simulink model "Expriment_Emotion"  (R2014a)
settings: Solver=FixedStepDiscrete  SolverMode=SingleTasking  StartTime=0.0  StopTime=inf  FixedStep=0.01  RelTol=1e-3
PostLoadFcn:
  | h_RPStest = RPStest;
model workspace (MAT data in the model file):
  gtest = 0
undefined symbols (not defined in the file or in its folder): avert, avert_freq_factor, avert_gaze_dirs_chance, avert_gaze_duration_factor, avert_head_frequency_factor, avert_head_speed, BML, BML1, BML2, bmlsL, bmlsM, bodyBusyFlag, clock, emotion_amount_factor, faceBusyFlag, fileID, GAZE_WIN, gazing, mut_freq_factor, mutual_gaze_duration_factor, P, pose_cat_chance, pose_chanc_factor, pose_chance_factor, pose_frequency_factor, pose_lean, pose_lean_flag, pose_space, pose_speed, pose_twitch, pr, serial, STATE_BEFORE, STATE_GO, STATE_OVER, STATE_READY, Stateflow
libraries: simulink x24, instrumentlib x6, realtime_pacer_lib x2, lib_affectiveChar_behavior x1, lib_affectiveChar_input x1
(part 6 of 6)

== matlab function Expriment_Emotion/facialExpr/facialExprGen/emotionBMLsLoop/loopInBmls ==
  data: i input double size=1 [1..]; arrAU input; eAmount input; arrBML output
function arrBML = fcn(i,arrAU,eAmount)
    %#codegen
    coder.extrinsic('sprintf');
    coder.extrinsic('strcat');
    
    %Maryam, 14-10-2015
    %'strcat' dimension 2  maximum size is 453,it was not possible to concat and send all bmls 
    %for one emotion together(used simulink for loop )    
    
    AU=arrAU(i);eA=eAmount(i);   
    c1 = countDigits(AU);c2 = countDigits(eA);

    str1 = sprintf('<?xml version=\"1.0\" ?><act><bml>');
    
    if(max(ceil(log10(abs(AU))),1)==1) %if AU is one-digit
        temp = sprintf('<face type=\"FACS\" side=\"BOTH\" au=\"%1d\"  start=\"0\" end=\"3\" amount=\"%0.1f\"/>',AU,eA); 
        temp2=strcat(str1,temp);
        str1=temp2;
    else      
        temp = sprintf('<face type=\"FACS\" side=\"BOTH\" au=\"%2d\"  start=\"0\" end=\"3\" amount=\"%0.1f\"/>',AU,eA);
        temp2=strcat(str1,temp);
        str1=temp2;
    end

    str2 = sprintf('</bml></act>');
    %n=length(arrAU);
    %mystr=blanks(arrAU(n));
    mystr=blanks(140+c1+c2);
    mystr = strcat (str1,str2);    
    arrBML = encStr2Arr(mystr);

== matlab function Expriment_Emotion/facialExpr/facialExprGen/forloop/makeBmlsFor ==
  data: i input double size=1 [1..]; arrAU input; eAmount input; arrBML1 output; arrBML2 output; arrBML3 output; arrBML4 output; arrBML5 output; arrBML6 output
function [arrBML1,arrBML2,arrBML3,arrBML4,arrBML5,arrBML6] = fcn(i,arrAU,eAmount)
    %#codegen
    coder.extrinsic('sprintf');
    coder.extrinsic('strcat');
    arrBML1=encStr2Arr('');arrBML2=encStr2Arr('');arrBML3=encStr2Arr('');
    arrBML4=encStr2Arr('');arrBML5=encStr2Arr('');arrBML6=encStr2Arr('');
    %Maryam, 14-10-2015
    %'strcat' dimension 2  maximum size is 453,it was not possible to concat and send all bmls 
    %for one emotion together(used simulink for loop )    
    
    AU=arrAU(i);eA=eAmount(i);   
    c1 = countDigits(AU);c2 = countDigits(eA);

    str1 = sprintf('<?xml version=\"1.0\" ?><act><bml>');
    
    if(max(ceil(log10(abs(AU))),1)==1) %if AU is one-digit
        temp = sprintf('<face type=\"FACS\" side=\"BOTH\" au=\"%1d\"  start=\"0\" ready=\"1\" stroke=\"2\"  relax=\"3\" end=\"4\" amount=\"%0.1f\"/>',AU,eA); 
        temp2=strcat(str1,temp);
        str1=temp2;
    else      
        temp = sprintf('<face type=\"FACS\" side=\"BOTH\" au=\"%2d\" start=\"0\" ready=\"1\" stroke=\"2\"  relax=\"3\" end=\"4\" amount=\"%0.1f\"/>',AU,eA);
        temp2=strcat(str1,temp);
        str1=temp2;
    end

    str2 = sprintf('</bml></act>');
    %n=length(arrAU);
    %mystr=blanks(arrAU(n));
    mystr=blanks(140+c1+c2);
    mystr = strcat (str1,str2);  
    if(i==1)
        arrBML1 = encStr2Arr(mystr);
    elseif(i==2)
        arrBML2 = encStr2Arr(mystr);
     elseif(i==3)
            arrBML3 = encStr2Arr(mystr);
     elseif(i==4)
            arrBML4 = encStr2Arr(mystr);
     elseif(i==5)
            arrBML5 = encStr2Arr(mystr);
     elseif(i==6)
            arrBML6 = encStr2Arr(mystr);
    end

== matlab function Expriment_Emotion/facialExpr/facialExprGen/matlabFuncIf/reset ==
  data: L input; u1 input; y output
function y = fcn(L,u1)
if(u1<=L)
    y= u1;
else
    y =1;
end

== matlab function Expriment_Emotion/facialExpr/facialExprGen/matlabFuncIf/displayBMLs ==
  data: e input; l input; i input double size=1 [1..]; bml input
function fcn(e,l,i,bml)
%#codegen
fprintf('%s','e:');fprintf('%f',e);
fprintf('%s','  ,L:');fprintf('%f',l);
fprintf('%s','  ,i:');fprintf('%f',i);
disp(decArr2Str(bml));

== matlab function Expriment_Emotion/facialExpr/facialExprGen/matlabFuncIf/plusOne ==
  data: y output; i input double size=1
function y  = iCheck(i)
%#codegen
    y=i+1;

== matlab function Expriment_Emotion/facialExpr/facialExprGen/matlabFuncIf/makeBmls ==
  data: i input double size=1 [1..]; arrAU input; eAmount input; arrBML output
function arrBML = fcn(i,arrAU,eAmount)
    %#codegen
    coder.extrinsic('sprintf');
    coder.extrinsic('strcat');
    
    %Maryam, 14-10-2015
    %'strcat' dimension 2  maximum size is 453,it was not possible to concat and send all bmls 
    %for one emotion together(used simulink for loop )    
    
    AU=arrAU(i);eA=eAmount(i);   
    c1 = countDigits(AU);c2 = countDigits(eA);

    str1 = sprintf('<?xml version=\"1.0\" ?><act><bml>');
    
    if(max(ceil(log10(abs(AU))),1)==1) %if AU is one-digit
        temp = sprintf('<face type=\"FACS\" side=\"BOTH\" au=\"%1d\"  start=\"0\" ready=\"1\" stroke=\"2\"  relax=\"300\" end=\"400\" amount=\"%0.1f\"/>',AU,eA); 
        temp2=strcat(str1,temp);
        str1=temp2;
    else      
        temp = sprintf('<face type=\"FACS\" side=\"BOTH\" au=\"%2d\" start=\"0\" ready=\"1\" stroke=\"2\"  relax=\"300\" end=\"400\" amount=\"%0.1f\"/>',AU,eA);
        temp2=strcat(str1,temp);
        str1=temp2;
    end

    str2 = sprintf('</bml></act>');
    %n=length(arrAU);
    %mystr=blanks(arrAU(n));
    mystr=blanks(142+c1+c2);
    mystr = strcat (str1,str2);    
    arrBML = encStr2Arr(mystr);

== matlab function Expriment_Emotion/facialExpr/facialExprGen/forloop1/displayBMLs ==
  data: e input; l input; i input double size=1 [1..]; bml input
function fcn(e,l,i,bml)
%#codegen
fprintf('%s','e:');fprintf('%f',e);
fprintf('%s','  ,L:');fprintf('%f',l);
fprintf('%s','  ,i:');fprintf('%f',i);
disp(decArr2Str(bml));

== matlab function Expriment_Emotion/facialExpr/facialExprGen/forloop1/makeBmls ==
  data: i input double size=1 [1..]; arrAU input; eAmount input; arrBML output
function arrBML = fcn(i,arrAU,eAmount)
    %#codegen
    coder.extrinsic('sprintf');
    coder.extrinsic('strcat');
    
    %Maryam, 14-10-2015
    %'strcat' dimension 2  maximum size is 453,it was not possible to concat and send all bmls 
    %for one emotion together(used simulink for loop )    
    
    AU=arrAU(i);eA=eAmount(i);   
    c1 = countDigits(AU);c2 = countDigits(eA);

    str1 = sprintf('<?xml version=\"1.0\" ?><act><bml>');
    
    if(max(ceil(log10(abs(AU))),1)==1) %if AU is one-digit
        temp = sprintf('<face type=\"FACS\" side=\"BOTH\" au=\"%1d\"  start=\"0\" ready=\"1\" stroke=\"2\"  relax=\"3\" end=\"4\" amount=\"%0.1f\"/>',AU,eA); 
        temp2=strcat(str1,temp);
        str1=temp2;
    else      
        temp = sprintf('<face type=\"FACS\" side=\"BOTH\" au=\"%2d\" start=\"0\" ready=\"1\" stroke=\"2\"  relax=\"3\" end=\"4\" amount=\"%0.1f\"/>',AU,eA);
        temp2=strcat(str1,temp);
        str1=temp2;
    end

    str2 = sprintf('</bml></act>');
    %n=length(arrAU);
    %mystr=blanks(arrAU(n));
    mystr=blanks(140+c1+c2);
    mystr = strcat (str1,str2);    
    arrBML = encStr2Arr(mystr);

== stateflow chart Expriment_Emotion/GazeFollowSubsystem/resetGazeTarget/createGazePawn ==
  state sendSBM(In2) [function]
  state stateCreatePawn
    entry:
    sendSBM(encStr2Arr('scene.getPawn(\"gazeTarget\").setPosition(SrVec(0,1.6,10))'));
  (default) -> stateCreatePawn
  data: In2 function_input double size=[1000 1]

== matlab function Expriment_Emotion/chack_E_Change1/checkNeutral ==
  data: notNeutral output double size=1; e input
function notNeutral = fcn(e)
%#codegen

if(e~=6)
    notNeutral=1;
else
    notNeutral=0;
end

== matlab function Expriment_Emotion/setPersonality ==
  data: extrovert input; personality output; neurotic input
function personality = fcn(extrovert,neurotic)
%#codegen
% 1 HEHN 2 LEHN 3 HELN 4 LELN
if(extrovert==1)
    if(neurotic==1)
        personality = 1;% 1 HEHN
    else 
        personality = 3;%HELN
    end
else
    if(neurotic==1)
        personality = 2;%LEHN
    else
        personality = 4;%LELN
    end
end

== matlab function Expriment_Emotion/EmotionSubsystem/calculateValenceArousal/HEHN_VA_Emo ==
  data: V input; e output double size=1; A input double
function e = fcn(V, A)

aVarTruthTableCondition_1 = false;
aVarTruthTableCondition_2 = false;
aVarTruthTableCondition_3 = false;
aVarTruthTableCondition_4 = false;
aVarTruthTableCondition_5 = false;
aVarTruthTableCondition_6 = false;
aVarTruthTableCondition_7 = false;
aVarTruthTableCondition_8 = false;


% 7-happy  2,1

aVarTruthTableCondition_1 = logical(V>10 && A<40 && A>10);

% 8-ex  1,2 AND 2,2

aVarTruthTableCondition_2 = logical(V>0 && A>40);

% 4-fear  -1,2 AND -2,2

aVarTruthTableCondition_3 = logical(V<0 && A>40);

% 3-frust  -2,1

aVarTruthTableCondition_4 = logical(V<-10 && A<40 && A>10);

% 6-pleased  2,-1

aVarTruthTableCondition_5 = logical(V>10 && A<-10 && A>-40);

% 5-calm  1,-2 AND 2,-2

aVarTruthTableCondition_6 = logical(V>0 && A<-40);

% 1-bored  -1,-2 AND -2,-2

aVarTruthTableCondition_7 = logical(V<0 && A<-40);

% 2-sad  -2,-1

aVarTruthTableCondition_8 = logical(V<-10 && A<-10 && A>-40);

if (aVarTruthTableCondition_1)
    aFcnTruthTableAction_1();
elseif (aVarTruthTableCondition_2)
    aFcnTruthTableAction_2();
elseif (aVarTruthTableCondition_3)
    aFcnTruthTableAction_3();
elseif (aVarTruthTableCondition_4)
    aFcnTruthTableAction_4();
elseif (aVarTruthTableCondition_5)
    aFcnTruthTableAction_5();
elseif (aVarTruthTableCondition_6)
    aFcnTruthTableAction_6();
elseif (aVarTruthTableCondition_7)
    aFcnTruthTableAction_7();
elseif (aVarTruthTableCondition_8)
    aFcnTruthTableAction_8();
else % Default
    aFcnTruthTableAction_5();
end

function aFcnTruthTableAction_1()

% happy

e=7;

function aFcnTruthTableAction_2()

% excited

e=8;

function aFcnTruthTableAction_3()

% fear

e=4;

function aFcnTruthTableAction_4()

% frustration

e=3;

function aFcnTruthTableAction_5()

% pleased

e=6;

function aFcnTruthTableAction_6()

% contempt

e=5;

function aFcnTruthTableAction_7()

% bored

e=1;

function aFcnTruthTableAction_8()

% sad

e=2;

== matlab function Expriment_Emotion/EmotionSubsystem/calculateValenceArousal/HELN_VA_Emo ==
  data: V input; e output double size=1; A input double
function e = fcn(V, A)

aVarTruthTableCondition_1 = false;
aVarTruthTableCondition_2 = false;
aVarTruthTableCondition_3 = false;
aVarTruthTableCondition_4 = false;
aVarTruthTableCondition_5 = false;
aVarTruthTableCondition_6 = false;
aVarTruthTableCondition_7 = false;
aVarTruthTableCondition_8 = false;


% 7-happy  2,1

aVarTruthTableCondition_1 = logical(V>10 && A<40 && A>10);

% 8-ex  1,2 AND 2,2

aVarTruthTableCondition_2 = logical(V>0 && A>40);

% 4-fear  -1,2 AND -2,2

aVarTruthTableCondition_3 = logical(V<0 && A>40);

% 3-frust  -2,1

aVarTruthTableCondition_4 = logical(V<-10 && A<40 && A>10);

% 6-idle  2,-1

aVarTruthTableCondition_5 = logical(V>10 && A<-10 && A>-40);

% 5-calm  1,-2 AND 2,-2

aVarTruthTableCondition_6 = logical(V>0 && A<-40);

% 1-bored  -1,-2 AND -2,-2

aVarTruthTableCondition_7 = logical(V<0 && A<-40);

% 2-sad  -2,-1

aVarTruthTableCondition_8 = logical(V<-10 && A<-10 && A>-40);

if (aVarTruthTableCondition_1)
    aFcnTruthTableAction_1();
elseif (aVarTruthTableCondition_2)
    aFcnTruthTableAction_2();
elseif (aVarTruthTableCondition_3)
    aFcnTruthTableAction_3();
elseif (aVarTruthTableCondition_4)
    aFcnTruthTableAction_4();
elseif (aVarTruthTableCondition_5)
    aFcnTruthTableAction_5();
elseif (aVarTruthTableCondition_6)
    aFcnTruthTableAction_6();
elseif (aVarTruthTableCondition_7)
    aFcnTruthTableAction_7();
elseif (aVarTruthTableCondition_8)
    aFcnTruthTableAction_8();
else % Default
    aFcnTruthTableAction_5();
end

function aFcnTruthTableAction_1()

% happy

e=7;

function aFcnTruthTableAction_2()

% excited

e=8;

function aFcnTruthTableAction_3()

% fear

e=4;

function aFcnTruthTableAction_4()

% frustration

e=3;

function aFcnTruthTableAction_5()

% idle

e=6;

function aFcnTruthTableAction_6()

% contempt

e=5;

function aFcnTruthTableAction_7()

% bored

e=1;

function aFcnTruthTableAction_8()

% sad

e=2;

== matlab function Expriment_Emotion/gazeInputArray/makeGazeArray ==
  data: r1 input; y output double size=[1,6]; r2 input; r3 input; r4 input; r5 input; r6 input
function y = fcn(r1,r2,r3,r4,r5,r6)
%#codegen
y=[0,0,0,0,0,0];
y(:,1) = floor(r1);
y(:,2) = floor(r2);
y(:,3) = floor(r3);
y(:,4) = floor(r4);
y(:,5) = floor(r5);
y(:,6) = floor(r6);

== matlab function Expriment_Emotion/EmotionSubsystem/calculateValenceArousal/LELN_VA_Emo ==
  data: V input; e output double size=1; A input double
function e = fcn(V, A)

aVarTruthTableCondition_1 = false;
aVarTruthTableCondition_2 = false;
aVarTruthTableCondition_3 = false;
aVarTruthTableCondition_4 = false;
aVarTruthTableCondition_5 = false;
aVarTruthTableCondition_6 = false;
aVarTruthTableCondition_7 = false;
aVarTruthTableCondition_8 = false;


% 7-happy  2,1

aVarTruthTableCondition_1 = logical(V>20 && A<40 && A>20);

% 8-ex  1,2 AND 2,2

aVarTruthTableCondition_2 = logical(V>0 && A>40);

% 4-fear  -1,2 AND -2,2

aVarTruthTableCondition_3 = logical(V<0 && A>40);

% 3-frust  -2,1

aVarTruthTableCondition_4 = logical(V<-20 && A<40 && A>20);

% 6-idle  2,-1

aVarTruthTableCondition_5 = logical(V>20 && A<-20 && A>-40);

% 5-calm  1,-2 AND 2,-2

aVarTruthTableCondition_6 = logical(V>0 && A<-40);

% 1-bored  -1,-2 AND -2,-2

aVarTruthTableCondition_7 = logical(V<0 && A<-40);

% 2-sad  -2,-1

aVarTruthTableCondition_8 = logical(V<-20 && A<-20 && A>-40);

if (aVarTruthTableCondition_1)
    aFcnTruthTableAction_1();
elseif (aVarTruthTableCondition_2)
    aFcnTruthTableAction_2();
elseif (aVarTruthTableCondition_3)
    aFcnTruthTableAction_3();
elseif (aVarTruthTableCondition_4)
    aFcnTruthTableAction_4();
elseif (aVarTruthTableCondition_5)
    aFcnTruthTableAction_5();
elseif (aVarTruthTableCondition_6)
    aFcnTruthTableAction_6();
elseif (aVarTruthTableCondition_7)
    aFcnTruthTableAction_7();
elseif (aVarTruthTableCondition_8)
    aFcnTruthTableAction_8();
else % Default
    aFcnTruthTableAction_5();
end

function aFcnTruthTableAction_1()

% happy

e=7;

function aFcnTruthTableAction_2()

% excited

e=8;

function aFcnTruthTableAction_3()

% fear

e=4;

function aFcnTruthTableAction_4()

% frustration

e=3;

function aFcnTruthTableAction_5()

% idle

e=6;

function aFcnTruthTableAction_6()

% contempt

e=5;

function aFcnTruthTableAction_7()

% bored

e=1;

function aFcnTruthTableAction_8()

% sad

e=2;

== matlab function Expriment_Emotion/EmotionSubsystem/calculateValenceArousal/HEHN_A ==
  data: a2 output double size=1; a1 input double size=1
function a2 = fcn(a1)

aVarTruthTableCondition_1 = false;
aVarTruthTableCondition_2 = false;



aVarTruthTableCondition_1 = logical(a1>10);


aVarTruthTableCondition_2 = logical(a1<-10);

if (aVarTruthTableCondition_1)
    aFcnTruthTableAction_1();
elseif (aVarTruthTableCondition_2)
    aFcnTruthTableAction_2();
else % Default
    aFcnTruthTableAction_3();
end

function aFcnTruthTableAction_1()


a2=a1;

function aFcnTruthTableAction_2()


a2=a1;

function aFcnTruthTableAction_3()


a2=0;

== matlab function Expriment_Emotion/EmotionSubsystem/calculateValenceArousal/LEHN_A ==
  data: a2 output double size=1; a1 input double size=1
function a2 = fcn(a1)

aVarTruthTableCondition_1 = false;
aVarTruthTableCondition_2 = false;



aVarTruthTableCondition_1 = logical(a1>25);


aVarTruthTableCondition_2 = logical(a1<-25);

if (aVarTruthTableCondition_1)
    aFcnTruthTableAction_1();
elseif (aVarTruthTableCondition_2)
    aFcnTruthTableAction_2();
else % Default
    aFcnTruthTableAction_3();
end

function aFcnTruthTableAction_1()


a2=a1;

function aFcnTruthTableAction_2()


a2=a1;

function aFcnTruthTableAction_3()


a2=0;

== matlab function Expriment_Emotion/EmotionSubsystem/calculateValenceArousal/HELN_A ==
  data: a2 output double size=1; a1 input double size=1
function a2 = fcn(a1)

aVarTruthTableCondition_1 = false;
aVarTruthTableCondition_2 = false;



aVarTruthTableCondition_1 = logical(a1>10);


aVarTruthTableCondition_2 = logical(a1<-10);

if (aVarTruthTableCondition_1)
    aFcnTruthTableAction_1();
elseif (aVarTruthTableCondition_2)
    aFcnTruthTableAction_2();
else % Default
    aFcnTruthTableAction_3();
end

function aFcnTruthTableAction_1()


a2=a1;

function aFcnTruthTableAction_2()


a2=a1;

function aFcnTruthTableAction_3()


a2=0;

== matlab function Expriment_Emotion/poseInputArray/makePoseArray ==
  data: r1 input; y output double size=[1,6]; r2 input; r3 input; r4 input; r5 input; r6 input
function y = fcn(r1,r2,r3,r4,r5,r6)
%#codegen
y=[0,0,0,0,0,0];
y(:,1) = floor(r1);
y(:,2) = floor(r2);
y(:,3) = floor(r3);
y(:,4) = floor(r4);
y(:,5) = floor(r5);
y(:,6) = floor(r6);

== matlab function Expriment_Emotion/EmotionSubsystem/calculateValenceArousal/HEHN plot ==
  data: v input; a input
function fcn(v,a)
%coder.extrinsic to bypass code generation
coder.extrinsic('fscanf')
coder.extrinsic('get_param');
% coder.extrinsic('importdata');

currentTime=get_param('Expriment_FacialExpr','SimulationTime');%use name of simulink proj

A = [v;a;currentTime];
fileID = fopen('HEHN_VA_table.txt','a');
fprintf(fileID,'%0.1f,%0.1f,%0.1f\r\n',A);
fclose(fileID);

% matrix = importdata('HEHN_VA_table.txt',','); 
% tri = delaunay(matrix(:,1),matrix(:,2));
% trisurf(tri,matrix(:,1),matrix(:,2),matrix(:,3))
% shading interp
% colorbar

%-----------------------------------------
% fileID = fopen('HEHN_VA_table.txt','r');
% formatSpec = '%1f\r %1f\r %1f\r\n';
% sizeA = [3 Inf];
% A = fscanf(fileID,formatSpec,sizeA)
% % A = A'
% fclose(fileID);

% x = zeros(100,2);y = zeros(100,2);
% filename = 'HEHN_VA_table.txt';
% delimiterIn = ' ';
% headerlinesIn = 1;
% A = importdata(filename,delimiterIn,headerlinesIn);

% fileID=fopen('HEHN_VA_table4.txt');
% s=textscan(fileID,'%d %d %d','headerlines',23);
% fclose(fileID);
% x=s{1}

== matlab function Expriment_Emotion/EmotionSubsystem/calculateValenceArousal/LEHN plot ==
  data: v input; a input
function fcn(v,a)
%coder.extrinsic to bypass code generation
coder.extrinsic('fscanf')
coder.extrinsic('get_param');
% coder.extrinsic('importdata');

currentTime=get_param('Expriment_FacialExpr','SimulationTime');%use name of simulink proj

A = [v;a;currentTime];

fileID = fopen('LEHN_VA_table.txt','a');
fprintf(fileID,'%0.1f,%0.1f,%0.1f\r\n',A);
fclose(fileID);

%use the following to draw the plot
%tmp_data = importdata('HEHN_VA_table.txt',','); 
%no need: x=tmp_data(:,1);y=tmp_data(:,2);z=tmp_data(:,3)
%matrix=tmp_data
%tri = delaunay(matrix(:,1),matrix(:,2));
%trisurf(tri,matrix(:,1),matrix(:,2),matrix(:,3))
%shading interp

%-----------------------------------------
% fileID = fopen('HEHN_VA_table.txt','r');
% formatSpec = '%1f\r %1f\r %1f\r\n';
% sizeA = [3 Inf];
% A = fscanf(fileID,formatSpec,sizeA)
% % A = A'
% fclose(fileID);

% x = zeros(100,2);y = zeros(100,2);
% filename = 'HEHN_VA_table.txt';
% delimiterIn = ' ';
% headerlinesIn = 1;
% A = importdata(filename,delimiterIn,headerlinesIn);

% fileID=fopen('HEHN_VA_table4.txt');
% s=textscan(fileID,'%d %d %d','headerlines',23);
% fclose(fileID);
% x=s{1}

== matlab function Expriment_Emotion/EmotionSubsystem/calculateValenceArousal/HELN plot ==
  data: v input; a input
function fcn(v,a)
%coder.extrinsic to bypass code generation
coder.extrinsic('fscanf')
coder.extrinsic('get_param');
% coder.extrinsic('importdata');

currentTime=get_param('Expriment_FacialExpr','SimulationTime');%use name of simulink proj

A = [v;a;currentTime];

fileID = fopen('HELN_VA_table.txt','a');
fprintf(fileID,'%0.1f,%0.1f,%0.1f\r\n',A);
fclose(fileID);

%use the following to draw the plot
%tmp_data = importdata('HEHN_VA_table.txt',','); 
%no need: x=tmp_data(:,1);y=tmp_data(:,2);z=tmp_data(:,3)
%matrix=tmp_data
%tri = delaunay(matrix(:,1),matrix(:,2));
%trisurf(tri,matrix(:,1),matrix(:,2),matrix(:,3))
%shading interp

%-----------------------------------------
% fileID = fopen('HEHN_VA_table.txt','r');
% formatSpec = '%1f\r %1f\r %1f\r\n';
% sizeA = [3 Inf];
% A = fscanf(fileID,formatSpec,sizeA)
% % A = A'
% fclose(fileID);

% x = zeros(100,2);y = zeros(100,2);
% filename = 'HEHN_VA_table.txt';
% delimiterIn = ' ';
% headerlinesIn = 1;
% A = importdata(filename,delimiterIn,headerlinesIn);

% fileID=fopen('HEHN_VA_table4.txt');
% s=textscan(fileID,'%d %d %d','headerlines',23);
% fclose(fileID);
% x=s{1}

== matlab function Expriment_Emotion/EmotionSubsystem/calculateValenceArousal/LELN plot ==
  data: v input; a input
function fcn(v,a)
%coder.extrinsic to bypass code generation
coder.extrinsic('fscanf')
coder.extrinsic('get_param');
% coder.extrinsic('importdata');

currentTime=get_param('Expriment_FacialExpr','SimulationTime');%use name of simulink proj

A = [v;a;currentTime];

fileID = fopen('LELN_VA_table.txt','a');
fprintf(fileID,'%0.1f,%0.1f,%0.1f\r\n',A);
fclose(fileID);

%use the following to draw the plot
%matrix = importdata('HEHN_VA_table.txt',','); 
%tri = delaunay(matrix(:,1),matrix(:,2));
%trisurf(tri,matrix(:,1),matrix(:,2),matrix(:,3))
%shading interp
%colorbar
%-----------------------------------------
% fileID = fopen('HEHN_VA_table.txt','r');
% formatSpec = '%1f\r %1f\r %1f\r\n';
% sizeA = [3 Inf];
% A = fscanf(fileID,formatSpec,sizeA)
% % A = A'
% fclose(fileID);

% x = zeros(100,2);y = zeros(100,2);
% filename = 'HEHN_VA_table.txt';
% delimiterIn = ' ';
% headerlinesIn = 1;
% A = importdata(filename,delimiterIn,headerlinesIn);

% fileID=fopen('HEHN_VA_table4.txt');
% s=textscan(fileID,'%d %d %d','headerlines',23);
% fclose(fileID);
% x=s{1}

== matlab function Expriment_Emotion/EmotionSubsystem/calculateValenceArousal/LELN_A ==
  data: a2 output double size=1; a1 input double size=1
function a2 = fcn(a1)

aVarTruthTableCondition_1 = false;
aVarTruthTableCondition_2 = false;



aVarTruthTableCondition_1 = logical(a1>25);


aVarTruthTableCondition_2 = logical(a1<-25);

if (aVarTruthTableCondition_1)
    aFcnTruthTableAction_1();
elseif (aVarTruthTableCondition_2)
    aFcnTruthTableAction_2();
else % Default
    aFcnTruthTableAction_3();
end

function aFcnTruthTableAction_1()


a2=a1;

function aFcnTruthTableAction_2()


a2=a1;

function aFcnTruthTableAction_3()


a2=0;

== matlab function Expriment_Emotion/EmotionSubsystem/calculateValenceArousal/HEHN_V ==
  data: v2 output double size=1; v1 input double size=1
function v2 = fcn(v1)

aVarTruthTableCondition_1 = false;
aVarTruthTableCondition_2 = false;



aVarTruthTableCondition_1 = logical(v1>10);


aVarTruthTableCondition_2 = logical(v1<-10);

if (aVarTruthTableCondition_1)
    aFcnTruthTableAction_1();
elseif (aVarTruthTableCondition_2)
    aFcnTruthTableAction_2();
else % Default
    aFcnTruthTableAction_3();
end

function aFcnTruthTableAction_1()


v2=v1;

function aFcnTruthTableAction_2()


v2=v1;

function aFcnTruthTableAction_3()


v2=0;

== matlab function Expriment_Emotion/EmotionSubsystem/calculateValenceArousal/LEHN_V ==
  data: v2 output double size=1; v1 input double size=1
function v2 = fcn(v1)

aVarTruthTableCondition_1 = false;
aVarTruthTableCondition_2 = false;



aVarTruthTableCondition_1 = logical(v1>25);


aVarTruthTableCondition_2 = logical(v1<-25);

if (aVarTruthTableCondition_1)
    aFcnTruthTableAction_1();
elseif (aVarTruthTableCondition_2)
    aFcnTruthTableAction_2();
else % Default
    aFcnTruthTableAction_3();
end

function aFcnTruthTableAction_1()


v2=v1;

function aFcnTruthTableAction_2()


v2=v1;

function aFcnTruthTableAction_3()


v2=0;

== matlab function Expriment_Emotion/EmotionSubsystem/calculateValenceArousal/HELN_V ==
  data: v2 output double size=1; v1 input double size=1
function v2 = fcn(v1)

aVarTruthTableCondition_1 = false;
aVarTruthTableCondition_2 = false;



aVarTruthTableCondition_1 = logical(v1>10);


aVarTruthTableCondition_2 = logical(v1<-10);

if (aVarTruthTableCondition_1)
    aFcnTruthTableAction_1();
elseif (aVarTruthTableCondition_2)
    aFcnTruthTableAction_2();
else % Default
    aFcnTruthTableAction_3();
end

function aFcnTruthTableAction_1()


v2=v1;

function aFcnTruthTableAction_2()


v2=v1;

function aFcnTruthTableAction_3()


v2=0;

== matlab function Expriment_Emotion/EmotionSubsystem/calculateValenceArousal/LELN_V ==
  data: v2 output double size=1; v1 input double size=1
function v2 = fcn(v1)

aVarTruthTableCondition_1 = false;
aVarTruthTableCondition_2 = false;



aVarTruthTableCondition_1 = logical(v1>25);


aVarTruthTableCondition_2 = logical(v1<-25);

if (aVarTruthTableCondition_1)
    aFcnTruthTableAction_1();
elseif (aVarTruthTableCondition_2)
    aFcnTruthTableAction_2();
else % Default
    aFcnTruthTableAction_3();
end

function aFcnTruthTableAction_1()


v2=v1;

function aFcnTruthTableAction_2()


v2=v1;

function aFcnTruthTableAction_3()


v2=0;

== stateflow chart Expriment_Emotion/CharacterControl/emotion_Behavior_Factors ==
  state init
    entry: mutual_gaze_duration_factor=1;avert_gaze_duration_factor=1;avert_head_frequency_factor=20;avert_head_speed=1;avert_gaze_dirs_chance=0;,avert_freq_factor=1;mut_freq_factor=1;
    pose_frequency_factor=20;pose_chanc_factor=1;pose_cat_chance=70;pose_lean=12;pose_speed=1;pose_lean_flag=0;pose_space=0;
  state wait
  state setBehavior
    entry:
    [mutual_gaze_duration_factor, avert_gaze_duration_factor,avert_head_frequency_factor,avert_head_speed,avert_gaze_dirs_chance,avert_freq_factor,mut_freq_factor]=sharedFunc.setGazeFactors(inV,inA,personality,personalityFlag,vaFlag,gazeArray);
    [pose_twitch,pose_frequency_factor,pose_chanc_factor,pose_cat_chance,pose_lean,pose_speed,pose_lean_flag,pose_space]=sharedFunc.setPoseFactors(inV,inA,personality,personalityFlag,vaFlag,poseArray,personalityChange);
  state sharedFunc [group]
  (default) -> init
  init -> wait
  wait -> setBehavior [order 2] : [vChange==1]
  wait -> setBehavior [order 1] : [aChange==1]
  setBehavior -> wait
  data: inA input double size=1; inV input double size=1; personality input; gazeArray input; aChange input; personalityFlag input; vaFlag input; avert_head_frequency_factor data_store_memory; avert_gaze_duration_factor data_store_memory; mutual_gaze_duration_factor data_store_memory; avert_head_speed data_store_memory; avert_gaze_dirs_chance data_store_memory; poseArray input; pose_lean data_store_memory; pose_speed data_store_memory; pose_lean_flag data_store_memory; pose_cat_chance data_store_memory; pose_frequency_factor data_store_memory; pose_chanc_factor data_store_memory; personalityChange input; avert_freq_factor data_store_memory; mut_freq_factor data_store_memory; pose_twitch data_store_memory; vChange input; pose_space data_store_memory

== matlab function Expriment_Emotion/CharacterControl/emotion_Behavior_Factors/sharedFunc ==
  data: v function_input double size=1; a function_input double size=1; mutDurFactor function_output double size=1; avertDurFactor function_output double size=1; avertHeadFreqFactor function_output double size=1; p function_input double size=1; pFlag function_input boolean size=1; vaFlag function_input boolean size=1; avertHeadSpeed function_output double size=1; gazeArr function_input double size=[1,6]; avertDirsChance function_output double size=1; avertFreqFactor function_output double size=1; mutFreqFactor function_output double size=1; poseTwitch function_output double size=1; poseFreqFactor function_output double size=1; poseChanceFactor function_output double size=1; poseCatChance function_output double size=1; poseLean function_output double size=1; v function_input double size=1; ar function_input double size=1; p function_input double size=1; pFlag function_input boolean size=1; vaFlag function_input boolean size=1; poseSpeed function_output double size=1; poseArr function_input double size=[1,6]; poseLeanFlag function_output double size=1; personalityChange function_input double size=1; poseSpace function_output double size=1
function [mutDurFactor,avertDurFactor,avertHeadFreqFactor,avertHeadSpeed,avertDirsChance,avertFreqFactor,mutFreqFactor]=setGazeFactors(v,a,p,pFlag,vaFlag,gazeArr)
    % Valence/Arousal: ref?
    %V+A+ (excite,happy):high mutual dur,head avert freq less,high freq of change btw mut/avert(MMMMMMMAAMMMMMAMMMA)
    %V-A+ (fear,frust): mid mut/avert,,head avert freq mid,high freq of change btw mut/avert(MMAAMMMAAMMAAAMMMAAAMA)
    %V+A- (idle, calm): mid mut/avert,head avert freq mid,low freq of change btw mut/avert(MMMMMMMAAAAAAMMMMMAAAAA)
    %V-A- (bored,sad):  avert dur more,,head avert freq more,,high freq of change btw mut/avert(AAAAAAMAAAAAAAAMAAAAA)
    %V+A+: v>0 & a>0,V-A+: v<0 & a>0,V+A-:v>0 & a<0,V-A-:v<0 & a<0

    %paper: Effects of Direct and Averted Gaze on the Perception of Facially Communicated Emotion
    % rate of approach-oriented dispositions (i.e., anger and joy) higher for direct relative gaze stimuli
    %avoidance-oriented dispositions (i.e., fear and sadness) would be higher for averted gaze faces.

    %russel, mehrabian circumplex:
    % v-mid,a-mid:approach;     v-mid,a+:avoid;       v-mid,a-:avoid
    % v+,a-mid:mid-approach;    v+,a+:high-approach;  v+,a-:low-approach
    % v-,a-mid:mid-avoid;        v-,a+:high-avoid;    v-,a-:low-avoid

    % marsella, emotional gaze:
    % a+:high blink, faster move

    %Saccadic reaction time is between 0.18sec and 0.22sec on average.Minimum intersaccadic interval ranges from 0.05sec to 0.1sec
    %smartbody DOF:magnitude:~btw 5'&12'->chanceO:btw 3&8->aveDur:btw 0.26sec&0.18sec --> 
    %simulation sample time is 0.001 so btw 26 and 18
    %magnitude=-6.9*log(chanceO/15.7) -->  -6.9*log(3/15.7)=11.4,-6.9*log(8/15.7)=4.6
    %chanceO=randArray(:,7)-->(3,8); 
    %avertDur=(25+2.5*magnitude)/2*factor;(same for mutual):btw(25+2.5*11.4)/2=26,(25+2.5*4.6)/2=18
    %randHeadChance=randi([1,1+round(randArray(3,5)/avert_head_frequency_factor)]);
 
    mutDurFactor=1; 
    avertDurFactor=1;  
    avertHeadFreqFactor=20;
    avertHeadSpeed=1;%1=normal, 2=fast&up,3=slow&down
    avertDirsChance=0;%not 1 & 2 is normal
    avertFreqFactor=1;
    mutFreqFactor=1;
    
    if(v>50 && a>50)%V+A+,high-approach,mutual alot
        mutDurFactor=mutDurFactor*2; % /2
        avertDurFactor=round(avertDurFactor*0.5);  % /2
        avertHeadFreqFactor=round(avertHeadFreqFactor/3);%high-approach:head not avert
        %avertHeadSpeed=2;%aroused fast
    
    elseif(v<-50 && a>50) %V-A+,high-avoid, avert alot
        mutDurFactor=round(mutDurFactor*0.5); % /2
        avertDurFactor=avertDurFactor*2; % /2
        avertHeadFreqFactor=avertHeadFreqFactor+30;%high-avoid:head avert alot
        %avertHeadSpeed=2;%fast
    
    elseif(v>50 && a<-50) %V+A- ,low-approach, mutual most
        mutDurFactor=round(mutDurFactor*1.5); %  /2
        avertDurFactor=round(avertDurFactor*0.75); %/2
        avertHeadFreqFactor=round(avertHeadFreqFactor/2);%approach:head not avert
        %avertHeadSpeed=1;%slow&down
    
    elseif(v<-50 && a<-50) %V-A-,  low-avoid, avert most
        mutDurFactor=round(mutDurFactor*0.75); %/2
        avertDurFactor=round(avertDurFactor*1.5);% /2
        avertHeadFreqFactor=avertHeadFreqFactor+20;%avoid:head avert alot
        %avertHeadSpeed=1;%slow&down
    end

== matlab function Expriment_Emotion/CharacterControl/emotion_Behavior_Factors/sharedFunc ==
function [poseTwitch,poseFreqFactor,poseChanceFactor,poseCatChance,poseLean,poseSpeed,poseLeanFlag,poseSpace] =setPoseFactors(v,ar,p,pFlag,vaFlag,poseArr,personalityChange)   
    poseCatChance=70;
    poseChanceFactor=1;
    poseFreqFactor=20;
    poseSpeed=1;%1=normal;2=fast; 3=slow;
    poseLean=12;
    poseTwitch=0;
    poseLeanFlag=0;
    poseSpace=0;
% marsella, emotional gaze:
% a+:faster move,body fw
    if(vaFlag==1)
        if( ar>50)%A+
             poseSpeed=2;%high arouse fast move
             poseLeanFlag=1;
             poseLean=13;%high aroused lean fw
        end
        if(ar<-50)%A-
             poseSpeed=3;%slow arouse slow move
             poseLeanFlag=1;
             poseLean=12;%low aroused lean back
        end
    end
